simulink model "lab12"  (R2024b)
settings: Solver=VariableStepAuto  StartTime=0.0  StopTime=10.0  RelTol=1e-3
settings Model: Creator=rares  LastModifiedBy=rares

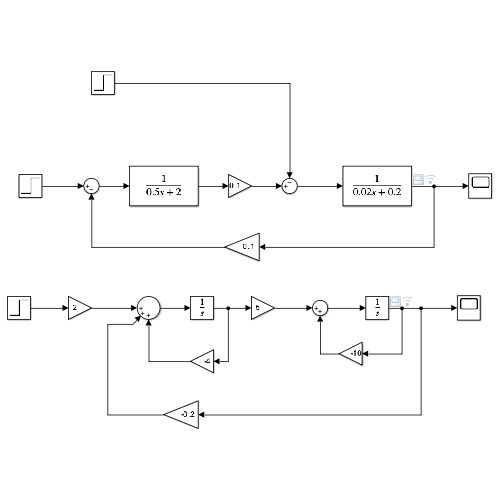
[thumbnail: Simulink's stored preview of the top-level diagram]
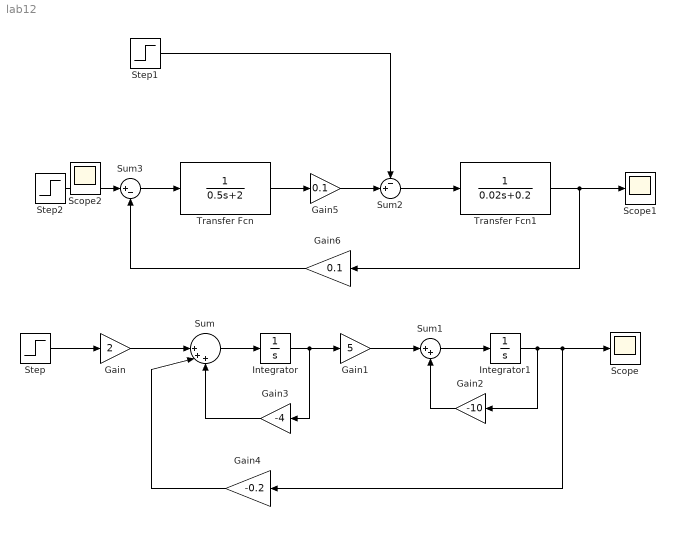
== system lab12 ==
  Gain : Gain  Gain=2
  Gain1 : Gain  Gain=5
  Gain2 : Gain  Gain=-10
  Gain3 : Gain  Gain=-4
  Gain4 : Gain  Gain=-0.2
  Gain5 : Gain  Gain=0.1
  Gain6 : Gain  Gain=0.1
  Integrator : Integrator
  Integrator1 : Integrator
  Scope : Scope
  Scope1 : Scope
  Step : Step  SampleTime=0
  Step1 : Step  SampleTime=0
  Step2 : Step  SampleTime=0
  Sum : Sum  Inputs=||+++
  Sum1 : Sum  Inputs=|++
  Sum2 : Sum  Inputs=-+|
  Sum3 : Sum  Inputs=|+-
  Transfer Fcn : TransferFcn  Denominator=[0.5 2]
  Transfer Fcn1 : TransferFcn  Denominator=[0.02 0.2]
  Scope2 : Scope
  wires:
  Step/1 -> Gain/1
  Gain/1 -> Sum/1
  Sum/1 -> Integrator/1
  Integrator/1 -> Gain3/1, Gain1/1
  Gain1/1 -> Sum1/1
  Sum1/1 -> Integrator1/1
  Integrator1/1 -> Gain2/1, Gain4/1, Scope/1
  Gain2/1 -> Sum1/2
  Gain3/1 -> Sum/3
  Gain4/1 -> Sum/2
  Step1/1 -> Sum2/1
  Gain5/1 -> Sum2/2
  Transfer Fcn/1 -> Gain5/1
  Sum3/1 -> Transfer Fcn/1
  Step2/1 -> Sum3/1
  Sum2/1 -> Transfer Fcn1/1
  Transfer Fcn1/1 -> Scope1/1, Gain6/1
  Gain6/1 -> Sum3/2
